simulink model "Implantation_Cmd_LQGI"  (R2022b)
settings: Solver=ode1  StartTime=0.0  StopTime=30  FixedStep=Te1  RelTol=1e-3  EnableMultiTasking=on
values from neighbouring files (symbols this model uses):
  A = [0 1;-Mb*g*Dm/Jp -Dp/Jp]    [InitCommande_Aero.m]    (also in apoio.m)
  B = [0; Dt*Kt/Jp]    [InitCommande_Aero.m]    (also in apoio.m = [0; Dt/Jp])
  C = [1 0]    [InitCommande_Aero.m]    (also in apoio.m)
  K_lqi = lqr(Aa, B1a, Q, R)    [InitCommande_Aero.m]
  Kw = Ka(1)    [InitCommande_Aero.m]    (also in matlab_variables_2_2.mat = 0.240350108962)
  Kz = Ka(2)    [InitCommande_Aero.m]    (also in matlab_variables_2_2.mat = 4.57892915652)
  L = place(Asys.', Csys.', p).'    [InitCommande_Aero.m]
  Te1 = 0.002    [InitCommande_Aero.m]    (also in matlab_variables_2_2.mat)
  Te2 = 0.02    [InitCommande_Aero.m]
libraries: quanser_aero x1, simulink_extras x1
settings Model: SimulationMode=external  ExtModeTrigDuration=50000  Creator=MLevis  LastModifiedBy=AERO3
settings SolverCC: AlgebraicLoopSolver=TrustRegion  PositivePriorityOrder=on
settings DataIOCC: SaveFormat=Array  DSMLogging=off  ReturnWorkspaceOutputs=off
settings DebuggingCC: SolverPrmCheckMsg=warning  UnconnectedInputMsg=warning  UnconnectedOutputMsg=warning  UnconnectedLineMsg=warning  SFUnexpectedBacktrackingDiag=warning  SFNoUnconditionalDefaultTransitionDiag=warning  SFExecutionAtInitializationDiag=none  SFMachineParentedDataDiag=warning  ArithmeticOperatorsInVariantConditions=warning
settings ModelReferenceCC: EnableRefExpFcnMdlSchedulingChecks=on  PropagateSignalLabelsOutOfModel=off
settings SFSimCC: SimUseLocalCustomCode=off  CustomCodeUndefinedFunction=UseInterfaceOnly
settings RTWCC: Description=QUARC Win64 Target Using Toolchain  SystemTargetFile=quarc_win64.tlc  TemplateMakefile=quarc_default_tmf  RTWUseLocalCustomCode=off  Toolchain=QUARC win64 | nmake (64-bit Windows)  BuildConfiguration=Faster Runs
settings CodeAppCC: StateflowObjectComments=on
settings STFCustomTargetCC: ConcurrentExecutionCompliant=on  GRTInterface=on  UseToolchainInfoCompliant=on  SystemTargetFile=quarc_win64.tlc
settings GRTTargetCC: TargetLangStandard=C89/C90 (ANSI)  ParMdlRefBuildCompliant=off  CompOptLevelCompliant=off  CombineOutputUpdateFcns=off  MatFileLogging=off  CPPClassGenCompliant=off  GRTInterface=on  ExtMode=on  ExtModeMexFile=quarc_comm
settings ConfigComp: CovMetricSettings=dw  CovSaveCumulativeToWorkspaceVar=on  CovSaveSingleToWorkspaceVar=on  CovExternalEMLEnable=off  CovSFcnEnable=off

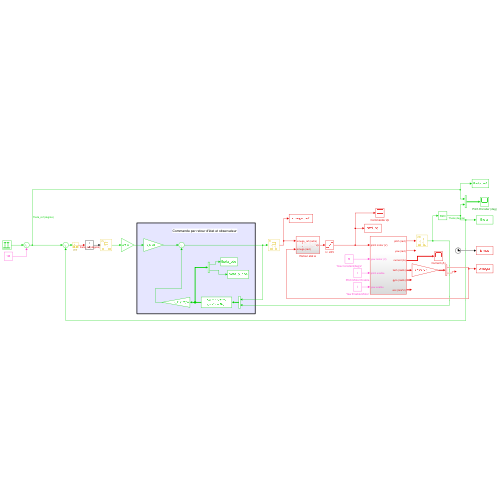
[thumbnail: Simulink's stored preview of the top-level diagram]
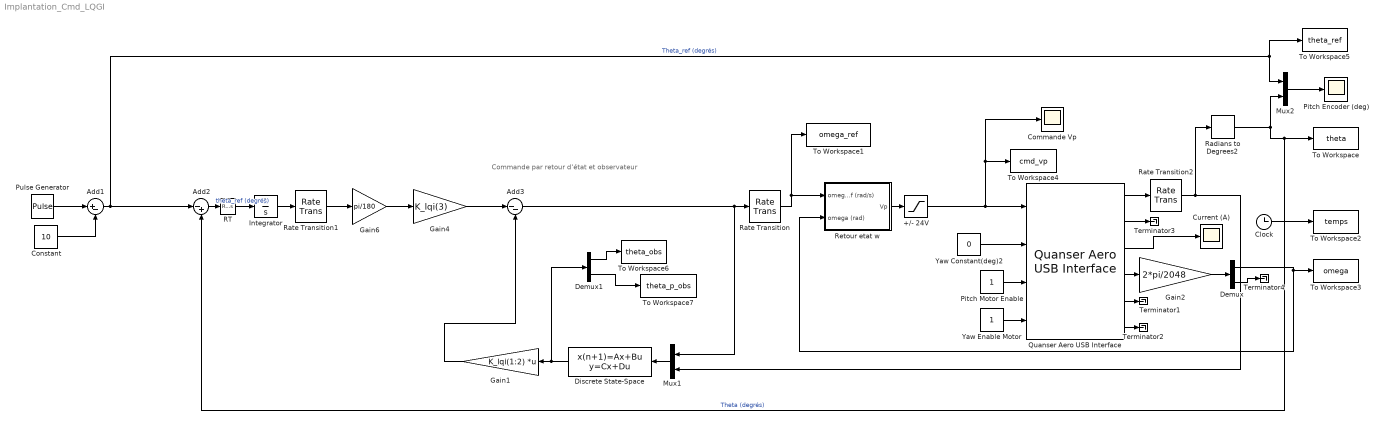
== system Implantation_Cmd_LQGI ==
  note: Commande par retour d'état et observateur
  +/- 24V : Saturate  UpperLimit=24  LowerLimit=-24
  Add1 : Sum  Inputs=|+-
  Add2 : Sum  Inputs=|-+
  Add3 : Sum  Inputs=|--
  Clock : Clock
  Commande Vp : Scope
  Constant : Constant  Value=10
  Current (A) : Scope
  Demux : Demux  Outputs=2
  Demux1 : Demux  Outputs=2
  Discrete State-Space : DiscreteStateSpace  A=eye(2)+(A-L*C)*Te2  B=[B L]*Te2  C=eye(2)  D=zeros(2,2)  SampleTime=Te2
  Gain1 : Gain  Gain=K_lqi(1:2)  Multiplication=Matrix(K*u)
  Gain2 : Gain  Gain=2*pi/2048
  Gain4 : Gain  Gain=K_lqi(3)
  Gain6 : Gain  Gain=pi/180
  Integrator : Integrator
  Mux1 : Mux  Inputs=2
  Mux2 : Mux  Inputs=2
  Pitch Encoder (deg) : Scope
  Pitch Motor Enable : Constant
  Pulse Generator : DiscretePulseGenerator  Amplitude=20  Period=ceil(20/Te2)  PulseWidth=ceil(10/Te2)  SampleTime=Te2
  Quanser Aero USB Interface : quanser_aero/Quanser Aero USB Interface  SystemSampleTime=-1  VariantActivationTime=update diagram  Latency=0  AutoFrameSizeCalculation=off
  RT : RateTransition  OutPortSampleTime=0.002
  Radians to Degrees2 : simulink_extras/Transformations/Radians to Degrees
  Rate Transition : RateTransition  OutPortSampleTime=Te1
  Rate Transition1 : RateTransition  OutPortSampleTime=Te2
  Rate Transition2 : RateTransition  OutPortSampleTime=Te2
  Retour etat w : Subsystem
  Terminator{1..4} (4 alike) : Terminator
  To Workspace : ToWorkspace  VariableName=theta  SampleTime=-1
      settings: Save2DSignal=2-D array (concatenate along first dimension)
  To Workspace1 : ToWorkspace  VariableName=omega_ref  SampleTime=-1
      settings: Save2DSignal=2-D array (concatenate along first dimension)
  To Workspace2 : ToWorkspace  VariableName=temps  SampleTime=-1
      settings: Save2DSignal=2-D array (concatenate along first dimension)
  To Workspace3 : ToWorkspace  VariableName=omega  SampleTime=-1
      settings: Save2DSignal=2-D array (concatenate along first dimension)
  To Workspace4 : ToWorkspace  VariableName=cmd_vp  SampleTime=-1
      settings: Save2DSignal=2-D array (concatenate along first dimension)
  To Workspace5 : ToWorkspace  VariableName=theta_ref  SampleTime=-1
      settings: Save2DSignal=2-D array (concatenate along first dimension)
  To Workspace6 : ToWorkspace  VariableName=theta_obs  SampleTime=-1
      settings: Save2DSignal=2-D array (concatenate along first dimension)
  To Workspace7 : ToWorkspace  VariableName=theta_p_obs  SampleTime=-1
      settings: Save2DSignal=2-D array (concatenate along first dimension)
  Yaw Constant(deg)2 : Constant  Value=0
  Yaw Enable Motor : Constant
  wires:
  Pitch Motor Enable/1 -> Quanser Aero USB Interface/3
  Yaw Enable Motor/1 -> Quanser Aero USB Interface/4
  +/- 24V/1 -> Quanser Aero USB Interface/1, Commande Vp/1, To Workspace4/1
  Quanser Aero USB Interface/3 -> Current (A)/1
  Quanser Aero USB Interface/4 -> Gain2/1
  Quanser Aero USB Interface/5 -> Terminator1/1
  Quanser Aero USB Interface/6 -> Terminator2/1
  Yaw Constant(deg)2/1 -> Quanser Aero USB Interface/2
  Radians to Degrees2/1 -> Mux2/2, Add2/2, To Workspace/1  "Theta (degrés)"
  Quanser Aero USB Interface/2 -> Terminator3/1
  Clock/1 -> To Workspace2/1
  Demux/1 -> Retour etat w/2(omega (rad)), To Workspace3/1
  Gain2/1 -> Demux/1
  Demux/2 -> Terminator4/1
  Add1/1 -> Add2/1, Mux2/1, To Workspace5/1  "Theta_ref (degrés)"
  Constant/1 -> Add1/2
  Pulse Generator/1 -> Add1/1
  Mux2/1 -> Pitch Encoder (deg)/1
  Rate Transition/1 -> Retour etat w/1(omega_ref (rad/s)), To Workspace1/1
  Retour etat w/1(Vp) -> +/- 24V/1
  Quanser Aero USB Interface/1 -> Rate Transition2/1
  Mux1/1 -> Discrete State-Space/1
  Demux1/1 -> To Workspace6/1
  Discrete State-Space/1 -> Demux1/1, Gain1/1
  Demux1/2 -> To Workspace7/1
  Gain4/1 -> Add3/1
  Gain1/1 -> Add3/2
  Rate Transition2/1 -> Radians to Degrees2/1, Mux1/2
  Add3/1 -> Mux1/1, Rate Transition/1
  Integrator/1 -> Rate Transition1/1
  Rate Transition1/1 -> Gain6/1
  Gain6/1 -> Gain4/1
  Add2/1 -> RT/1
  RT/1 -> Integrator/1  "theta_ref (degrés)"

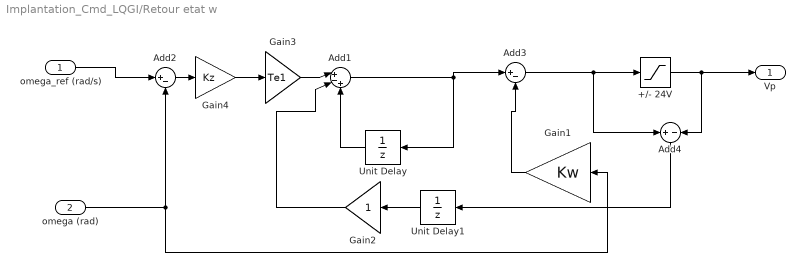
== system Implantation_Cmd_LQGI/Retour etat w ==
  omega_ref (rad/s) : Inport
  omega (rad) : Inport  Port=2
  +/- 24V : Saturate  UpperLimit=24  LowerLimit=-24
  Add1 : Sum  Inputs=|+-+
  Add2 : Sum  Inputs=|+-
  Add3 : Sum  Inputs=|+-
  Add4 : Sum  Inputs=+-
  Gain1 : Gain  Gain=Kw
  Gain2 : Gain
  Gain3 : Gain  Gain=Te1
  Gain4 : Gain  Gain=Kz
  Unit Delay : UnitDelay  SampleTime=Te1  HasFrameUpgradeWarning=on
  Unit Delay1 : UnitDelay  SampleTime=Te1  HasFrameUpgradeWarning=on
  Vp : Outport  VectorParamsAs1DForOutWhenUnconnected=off
  wires:
  omega_ref (rad/s)/1 -> Add2/1
  Add2/1 -> Gain4/1
  omega (rad)/1 -> Add2/2, Gain1/1
  Gain1/1 -> Add3/2
  Add3/1 -> Add4/1, +/- 24V/1
  Gain3/1 -> Add1/1
  +/- 24V/1 -> Add4/2, Vp/1
  Gain4/1 -> Gain3/1
  Add1/1 -> Unit Delay/1, Add3/1
  Add4/1 -> Unit Delay1/1
  Unit Delay/1 -> Add1/3
  Gain2/1 -> Add1/2
  Unit Delay1/1 -> Gain2/1
